simulink model "recursive_estimation"  (R2023a)
settings: Solver=FixedStepAuto  StartTime=start_time  StopTime=stop_time  FixedStep=sample_time  RelTol=1e-3
values from neighbouring files (symbols this model uses):
  A = [1, a]    [example12.m]
  B = b    (= 0.5)    [example12.m]
  C = [1, c]    [example12.m]
  mean_e = 0    [example12.m]    (also in example14.m; example15.m)
  P0 = 100 * eye(3)    [example12.m]    (also in example14.m = 0.01 * eye(2); example15.m = 100 * eye(2); example16.m = 0.01)
  sample_time = 1    [example12.m]    (also in example14.m; example15.m; example16.m)
  seed_e = 6    [example12.m]    (also in example14.m = i; example15.m = 2)
  std_e = 0.5    [example12.m]    (also in example14.m; example15.m)
  theta0 = zeros(3,1)    [example12.m]    (also in example14.m = Theta(:,i); example15.m = zeros(2,1); example16.m = zeros(n_phi, 1))
settings Model: Creator=Beigi  LastModifiedBy=Mmoha

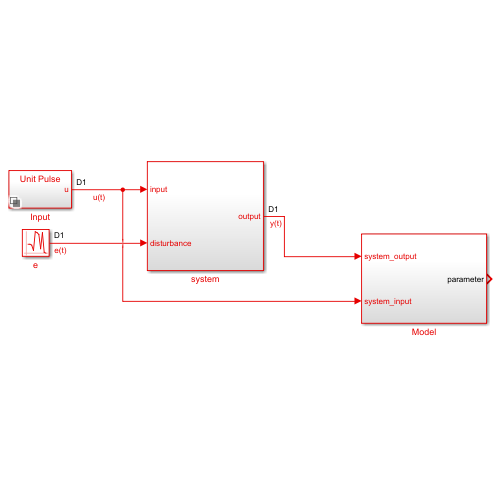
[thumbnail: Simulink's stored preview of the top-level diagram]
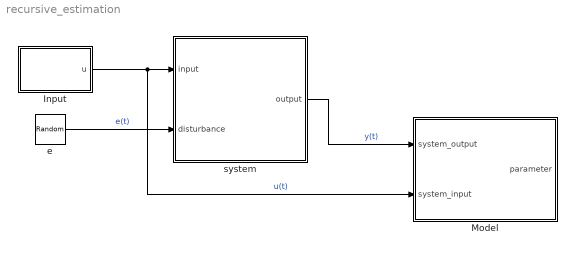
== system recursive_estimation ==
  Input : Subsystem  Variant=on  VariantControlMode=label  VariantControl=Choice  LabelModeActiveChoice=unit_pulse
  Model : Subsystem
  e : RandomNumber  Mean=mean_e  Variance=std_e^2  Seed=seed_e  SampleTime=sample_time
  system : Subsystem
  wires:
  e/1 -> system/2(disturbance)  "e(t)"
  Input/1(u) -> Model/2(system_input), system/1(input)  "u(t)"
  system/1(output) -> Model/1(system_output)  "y(t)"

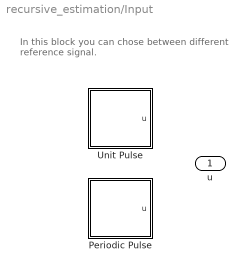
== system recursive_estimation/Input ==
  note: In this block you can chose between different
      | reference signal.
  Periodic Pulse : Subsystem  VariantControl=periodic_pulse
  Unit Pulse : Subsystem  VariantControl=unit_pulse
  u : Outport

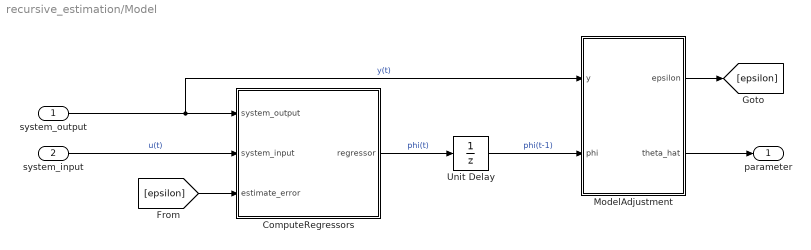
== system recursive_estimation/Model ==
  system_output : Inport
  system_input : Inport  Port=2
  ComputeRegressors : Subsystem  Variant=on  VariantControlMode=label  VariantControl=Choice  LabelModeActiveChoice=Choice
  ModelAdjustment : Subsystem
  Unit Delay : UnitDelay  SampleTime=-1  HasFrameUpgradeWarning=on
  parameter : Outport
  wires:
  system_output/1 -> ModelAdjustment/1(y), ComputeRegressors/1(system_output)  "y(t)"
  system_input/1 -> ComputeRegressors/2(system_input)  "u(t)"
  ComputeRegressors/1(regressor) -> Unit Delay/1  "phi(t)"
  Unit Delay/1 -> ModelAdjustment/2(phi)  "phi(t-1)"
  ModelAdjustment/1(epsilon) -> [epsilon]
  [epsilon] -> ComputeRegressors/3(estimate_error)
  ModelAdjustment/2(theta_hat) -> parameter/1

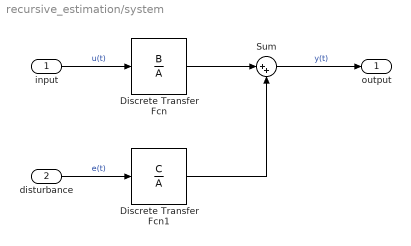
== system recursive_estimation/system ==
  input : Inport
  disturbance : Inport  Port=2
  Discrete Transfer Fcn : DiscreteTransferFcn  Numerator=B  Denominator=A
  Discrete Transfer Fcn1 : DiscreteTransferFcn  Numerator=C  Denominator=A
  Sum : Sum  Inputs=|++
  output : Outport
  wires:
  disturbance/1 -> Discrete Transfer Fcn1/1  "e(t)"
  input/1 -> Discrete Transfer Fcn/1  "u(t)"
  Discrete Transfer Fcn/1 -> Sum/1
  Discrete Transfer Fcn1/1 -> Sum/2
  Sum/1 -> output/1  "y(t)"

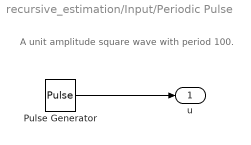
== system recursive_estimation/Input/Periodic Pulse ==
  note: A unit amplitude square wave with period 100.
  Pulse Generator : DiscretePulseGenerator  PulseType=Time based  Period=100  PulseWidth=50
  u : Outport
  wires:
  Pulse Generator/1 -> u/1

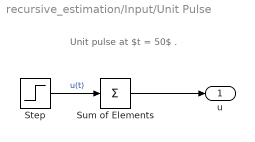
== system recursive_estimation/Input/Unit Pulse ==
  note: Unit pulse at $t = 50$ .
  Step : Step  Time=[50 51]  After=[1 -1]  SampleTime=sample_time
  Sum of Elements : Sum  Inputs=+
  u : Outport
  wires:
  Step/1 -> Sum of Elements/1  "u(t)"
  Sum of Elements/1 -> u/1

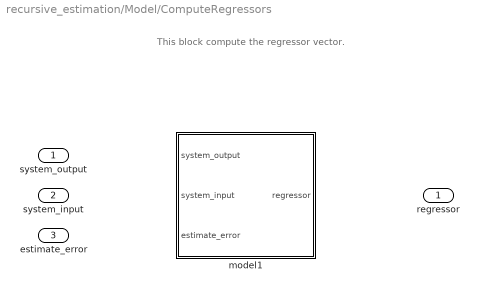
== system recursive_estimation/Model/ComputeRegressors ==
  note: This block compute the regressor vector.
  system_output : Inport
  system_input : Inport  Port=2
  estimate_error : Inport  Port=3
  model1 : Subsystem  VariantControl=Choice
  regressor : Outport

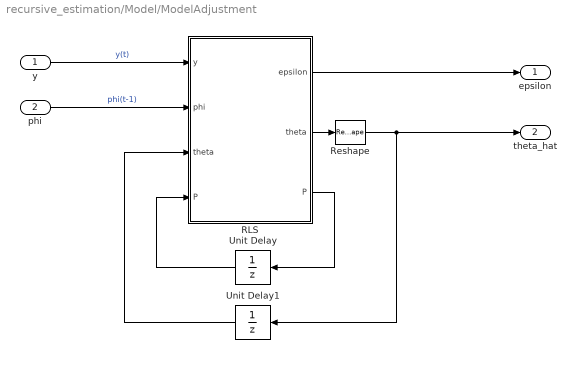
== system recursive_estimation/Model/ModelAdjustment ==
  y : Inport
  phi : Inport  Port=2
  RLS : MATLAB Function  TreatAsAtomicUnit=on
  Reshape : Reshape  OutputDimensionality=Column vector (2-D)
  Unit Delay : UnitDelay  InitialCondition=P0  SampleTime=-1  HasFrameUpgradeWarning=on
  Unit Delay1 : UnitDelay  InitialCondition=theta0  SampleTime=-1  HasFrameUpgradeWarning=on
  epsilon : Outport
  theta_hat : Outport  Port=2
  wires:
  phi/1 -> RLS/2(phi)  "phi(t-1)"
  RLS/3(P) -> Unit Delay/1
  Unit Delay/1 -> RLS/4("P ")
  Unit Delay1/1 -> RLS/3("theta ")
  RLS/2(theta) -> Reshape/1
  y/1 -> RLS/1(y)  "y(t)"
  Reshape/1 -> Unit Delay1/1, theta_hat/1
  RLS/1(epsilon) -> epsilon/1

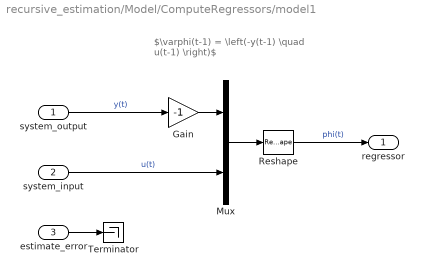
== system recursive_estimation/Model/ComputeRegressors/model1 ==
  note: $\varphi(t-1) = \left(-y(t-1) \quad u(t-1) \right)$
  system_output : Inport
  system_input : Inport  Port=2
  estimate_error : Inport  Port=3
  Gain : Gain  Gain=-1
  Mux : Mux  Inputs=2
  Reshape : Reshape  OutputDimensionality=Column vector (2-D)
  Terminator : Terminator
  regressor : Outport
  wires:
  estimate_error/1 -> Terminator/1
  system_output/1 -> Gain/1  "y(t)"
  system_input/1 -> Mux/2  "u(t)"
  Gain/1 -> Mux/1
  Mux/1 -> Reshape/1
  Reshape/1 -> regressor/1  "phi(t)"

== matlab function recursive_estimation/Model/ModelAdjustment/RLS ==
  data: y input; phi input; epsilon output; theta input; P input; theta output; P output
function [epsilon,theta,P] = fcn(y,phi,theta,P)
epsilon = y - phi' * theta;
P = P - P * phi / ( 1 + phi' * P * phi ) * phi' * P;
theta = theta + P * phi * epsilon;
